simulink model "sampleModel1928_2_sub_sub"  (R2023a)
settings: Solver=VariableStepAuto  StartTime=0.0  StopTime=10.0  RelTol=1e-3
libraries: hdlsllib x7, simulink x2
settings Model: Creator=user1  LastModifiedBy=user1

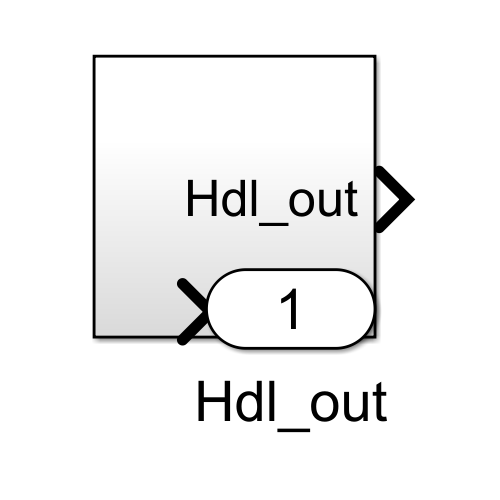
[thumbnail: Simulink's stored preview of the top-level diagram]
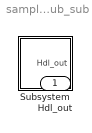
== system sampleModel1928_2_sub_sub ==
  Subsystem : Subsystem
  Hdl_out : Outport  OutDataTypeStr=uint8

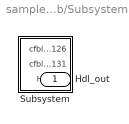
== system sampleModel1928_2_sub_sub/Subsystem ==
  Subsystem : Subsystem
  Hdl_out : Outport  OutDataTypeStr=uint8

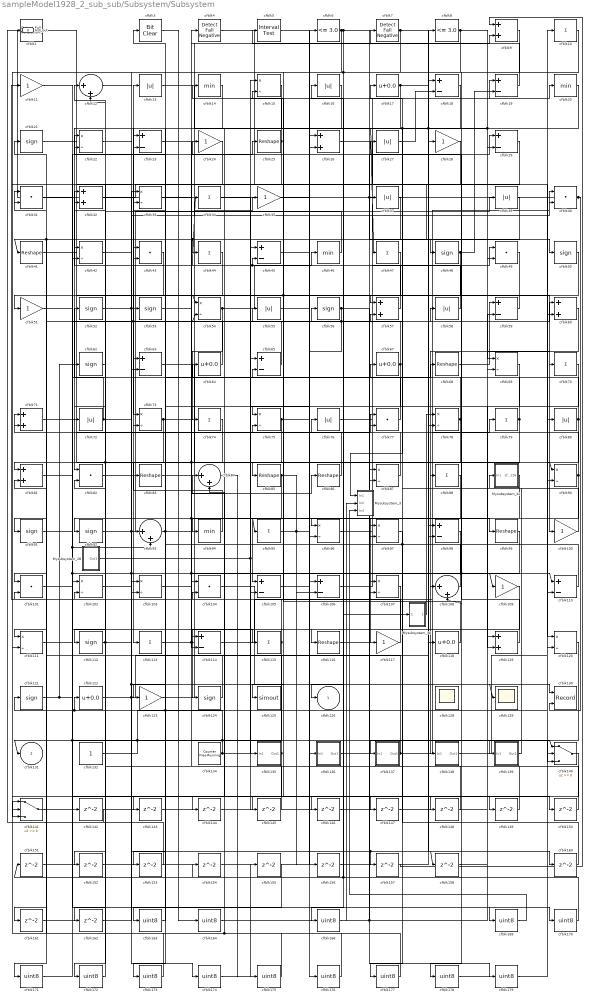
== system sampleModel1928_2_sub_sub/Subsystem/Subsystem ==
  Mysubsystem_28 : Subsystem  TreatAsAtomicUnit=on  RTWFcnName=Mysubsystem_28
      settings: RTWFcnNameOpts=User specified  RTWFileNameOpts=Use function name
  Mysubsystem_3 : Subsystem  TreatAsAtomicUnit=on  RTWFcnName=Mysubsystem_3
      settings: RTWFcnNameOpts=User specified  RTWFileNameOpts=Use function name
  Mysubsystem_38 : Subsystem  TreatAsAtomicUnit=on  RTWFcnName=Mysubsystem_38
      settings: RTWFcnNameOpts=User specified  RTWFileNameOpts=Use function name
  Mysubsystem_42 : Subsystem  TreatAsAtomicUnit=on  RTWFcnName=Mysubsystem_42
      settings: RTWFcnNameOpts=User specified  RTWFileNameOpts=Use function name
  cfblk1 : hdlsllib/Logic and Bit Operations/Detect Fall Nonpositive  vinit=0  OutDataTypeStr=uint8
  cfblk{10,34,44,47,70,74,79,88,95,113,115} (11 alike) : Sum  Inputs=+  OutDataTypeStr=uint8
  cfblk{11,24,28,35,51,100,109,117,123} (9 alike) : Gain  OutDataTypeStr=uint8
  cfblk{31,40,43,49,77,82,101,104} (8 alike) : DotProduct  OutDataTypeStr=uint8
  cfblk{15,22,33,42,54,69,73,75,78,87,90,96..97,102..103,107,111,120} (18 alike) : Product  Inputs=*/  OutDataTypeStr=uint8  RndMeth=Zero  SaturateOnIntegerOverflow=on
  cfblk{18..19,23,29,45,59,63,65,98,105..106,110,114} (13 alike) : Sum  Inputs=+-  OutDataTypeStr=uint8
  cfblk{12,84,93,108} (4 alike) : Sum  Inputs=|++  OutDataTypeStr=uint8
  cfblk{21,48,50,52..53,56,62,91..92,112,121,124} (12 alike) : Signum
  cfblk{25,41,68,83,85..86,99,116} (8 alike) : Reshape
  cfblk{17,64,67,118,122} (5 alike) : Bias  Bias=0.0  SaturateOnIntegerOverflow=off
  cfblk{9,26,32,57,60,71,81,119} (8 alike) : Sum  OutDataTypeStr=uint8
  cfblk125 : ToWorkspace  VariableName=simout  SaveFormat=Timeseries  SampleTime=-1
  cfblk128 : Scope
      settings: Floating=on
  cfblk129 : Scope
  cfblk{13,16,27,37,39,55,58,72,76,80} (10 alike) : Abs  OutDataTypeStr=uint8  SaturateOnIntegerOverflow=off
  cfblk130 : Record  FileSettingsInternal="{\"entries\":[{\"content\":{\"excelSettings\":{\"content\":{},\"type\":\"Streamout.ExcelSettings\"}},\"type\":\"Streamout.FileSettingStorage\",\"uuid\":\"\"}],\"packageUris\":[\"http:\\/\\/schema.mathworks.com\\/mf0\\/streamout_blocks\\/R2020a\"],\"version\":\"1.0\"}"  Layout=[1 1]  SignalsInternal="{\"entries\":[{\"content\":{\"signals\":[{\"content\":{\"blockPath\":[],\"dimensions\":[1],\"domain\":\"\",\"lineColor\":\"#a2142f\",\"plots\":[1],\"port\":1,\"signalID\":52207,\"signalName\":\"cfblk34\"},\"type\":\"RecordBlkView.Signal\",\"uuid\":\"\"},{\"content\":{\"blockPath\":[],\"dimensions\":[1],\"domain\":\"\",\"lineColor\":\"#139fff\",\"plots\":[1],\"port\":2,\"signalID\":52210,\"signalName\":\"cfblk40\"},\"type\":\"RecordBlkView.Signal\",\"uuid\":\"\"}]},\"type\":\"RecordBlkView.InputSignals\",\"uuid\":\"\"}],\"packageUris\":[\"http:\\/\\/schema.mathworks.com\\/mf0\\/streamout_blocks\\/R2020a\"],\"version\":\"1.0\"}"  VisualizationBindings="{\"xyplotplugin\":{\"info\":[{\"series\":[{\"bindingParametersList\":[{\"parameter\":\"X-Axis\",\"signalID\":52207,\"signalName\":\"cfblk34\"},{\"parameter\":\"Y-Axis\",\"signalID\":52210,\"signalName\":\"cfblk40\"}],\"seriesID\":26218}],\"subplotID\":1}]}}"  CompatibilityTag=XY  st=-1
  cfblk132 : Constant  OutDataTypeStr=uint8  SampleTime=-1
  cfblk134 : hdlsllib/Sources/Counter Free-Running  NumBits=16  tsamp=-1
  cfblk135 : Subsystem
      settings: LibrarySourceBlock=|
      | hdlsllib/Ports &
      | Subsystems/Subsystem
  cfblk136 : Subsystem
      settings: LibrarySourceBlock=|
      | hdlsllib/Ports &
      | Subsystems/Subsystem
  cfblk137 : Subsystem
      settings: LibrarySourceBlock=|
      | hdlsllib/Ports &
      | Subsystems/Subsystem
  cfblk138 : Subsystem
      settings: LibrarySourceBlock=|
      | hdlsllib/Ports &
      | Subsystems/Subsystem
  cfblk139 : Subsystem
      settings: LibrarySourceBlock=|
      | hdlsllib/Ports &
      | Subsystems/Subsystem
  cfblk{14,20,46,94} (4 alike) : MinMax  OutDataTypeStr=uint8
  cfblk140 : Switch  OutDataTypeStr=uint8  SaturateOnIntegerOverflow=off  InputSameDT=off
  cfblk141 : Switch  OutDataTypeStr=uint8  SaturateOnIntegerOverflow=off  InputSameDT=off
  cfblk{142..158,160..162} (20 alike) : Delay  SampleTime=1
  cfblk{163..164,166,169..179} (14 alike) : DataTypeConversion  OutDataTypeStr=uint8  SaturateOnIntegerOverflow=off  RndMeth=Floor
  cfblk3 : simulink/Logic and Bit Operations/Bit Clear  iBit=0
      settings: LibrarySourceBlock=|
      | hdlsllib/Logic and Bit
      | Operations/Bit Clear
  cfblk4 : hdlsllib/Logic and Bit Operations/Detect Fall Negative  vinit=0  OutDataTypeStr=uint8
  cfblk5 : hdlsllib/Logic and Bit Operations/Interval Test  IntervalClosedRight=on  uplimit=0.5  IntervalClosedLeft=on  lowlimit=-0.5  OutDataTypeStr=uint8
  cfblk6 : hdlsllib/Logic and Bit Operations/Compare To Constant  relop=<=  const=3.0  OutDataTypeStr=uint8
  cfblk7 : hdlsllib/Logic and Bit Operations/Detect Fall Negative  vinit=0  OutDataTypeStr=uint8
  cfblk8 : hdlsllib/Logic and Bit Operations/Compare To Constant  relop=<=  const=3.0  OutDataTypeStr=uint8
  cfblk126 : Outport  OutDataTypeStr=uint8  VectorParamsAs1DForOutWhenUnconnected=off
  cfblk131 : Outport  Port=2  OutDataTypeStr=uint8  VectorParamsAs1DForOutWhenUnconnected=off
  Hdl_out : Outport  Port=3  OutDataTypeStr=uint8
  wires:
  Mysubsystem_42/1(cfblk126) -> cfblk126/1
  cfblk139/1(Out1) -> Mysubsystem_42/1(In1)
  Mysubsystem_38/1(Out1) -> cfblk78/1
  Mysubsystem_28/1(Out1) -> cfblk106/1, cfblk135/1(In1)
  cfblk169/1 -> Mysubsystem_3/3(In3)
  cfblk166/1 -> Mysubsystem_3/2(In2)
  cfblk179/1 -> cfblk10/1
  cfblk178/1 -> cfblk120/2
  cfblk10/1 -> cfblk178/1
  cfblk177/1 -> cfblk84/2
  cfblk120/1 -> cfblk177/1
  cfblk176/1 -> cfblk84/1
  cfblk5/1 -> cfblk176/1
  cfblk175/1 -> cfblk154/1, cfblk121/1
  cfblk174/1 -> cfblk155/1
  cfblk42/1 -> cfblk174/1
  cfblk173/1 -> cfblk141/1
  cfblk155/1 -> cfblk173/1
  cfblk172/1 -> cfblk102/2
  cfblk62/1 -> cfblk172/1
  cfblk171/1 -> cfblk102/1
  cfblk170/1 -> cfblk151/1, cfblk76/1
  cfblk164/1 -> cfblk69/2, cfblk87/2
  cfblk163/1 -> cfblk3/1
  cfblk140/1 -> cfblk163/1
  cfblk162/1 -> cfblk33/1
  cfblk161/1 -> cfblk103/2
  cfblk160/1 -> cfblk57/2
  cfblk158/1 -> cfblk59/2
  cfblk157/1 -> cfblk9/1
  cfblk156/1 -> cfblk97/2
  cfblk154/1 -> cfblk98/2
  cfblk153/1 -> cfblk31/2
  cfblk152/1 -> cfblk26/2
  cfblk151/1 -> cfblk93/1
  cfblk150/1 -> cfblk87/1
  cfblk105/1 -> cfblk150/1
  cfblk149/1 -> cfblk104/1
  cfblk148/1 -> cfblk82/2
  cfblk147/1 -> cfblk18/1
  cfblk11/1 -> cfblk147/1
  cfblk146/1 -> cfblk119/1
  cfblk145/1 -> cfblk65/1
  cfblk107/1 -> cfblk145/1
  cfblk144/1 -> cfblk45/1
  cfblk143/1 -> cfblk15/1
  cfblk142/1 -> cfblk1/1
  cfblk111/1 -> cfblk142/1
  cfblk45/1 -> cfblk97/1
  cfblk54/1 -> cfblk46/1, cfblk74/1
  cfblk20/1 -> cfblk83/1, cfblk29/2
  cfblk35/1 -> cfblk99/1
  cfblk115/1 -> cfblk101/2, cfblk161/1
  cfblk116/1 -> cfblk68/1
  cfblk104/1 -> cfblk136/1(In1)
  cfblk88/1 -> cfblk107/1
  cfblk82/1 -> cfblk26/1
  cfblk46/1 -> cfblk22/1
  cfblk110/1 -> cfblk27/1, cfblk22/2
  cfblk124/1 -> cfblk71/2
  cfblk33/1 -> cfblk96/1, cfblk90/1
  cfblk53/1 -> cfblk114/1
  cfblk77/1 -> cfblk16/1
  cfblk22/1 -> cfblk107/2, cfblk148/1
  cfblk25/1 -> cfblk111/2, cfblk14/1
  cfblk99/1 -> cfblk108/2, cfblk114/2
  cfblk55/1 -> cfblk108/1
  cfblk59/1 -> cfblk57/1
  cfblk73/1 -> cfblk118/1, cfblk91/1
  cfblk109/1 -> cfblk124/1
  cfblk95/1 -> cfblk6/1, cfblk156/1
  cfblk49/1 -> cfblk54/1, cfblk85/1
  cfblk135/1(Out1) -> cfblk141/2, cfblk12/2
  cfblk3/1 -> cfblk164/1
  cfblk121/1 -> cfblk67/1, cfblk62/1
  cfblk67/1 -> cfblk43/2, cfblk153/1
  cfblk138/1(Out1) -> cfblk110/2
  cfblk84/1 -> cfblk175/1
  cfblk13/1 -> cfblk49/2
  cfblk63/1 -> cfblk98/1
  cfblk26/1 -> cfblk69/1
  cfblk24/1 -> cfblk123/1
  cfblk39/1 -> cfblk42/2, cfblk44/1
  cfblk80/1 -> cfblk23/2, cfblk90/2
  cfblk37/1 -> cfblk41/1, cfblk81/1
  cfblk44/1 -> cfblk72/1
  cfblk117/1 -> cfblk104/2
  cfblk112/1 -> cfblk53/1, cfblk12/1
  cfblk23/1 -> cfblk95/1, cfblk105/2
  cfblk50/1 -> cfblk101/1
  cfblk60/1 -> cfblk88/1
  cfblk132/1 -> cfblk140/1, cfblk80/1
  cfblk70/1 -> cfblk94/1
  cfblk118/1 -> cfblk65/2
  cfblk8/1 -> cfblk63/2, cfblk70/1
  cfblk1/1 -> cfblk103/1
  cfblk90/1 -> cfblk56/1, cfblk162/1
  cfblk103/1 -> cfblk9/2, cfblk109/1
  cfblk68/1 -> cfblk59/1
  cfblk100/1 -> cfblk17/1
  cfblk19/1 -> cfblk5/1
  cfblk136/1(Out1) -> cfblk37/1, cfblk29/1
  cfblk9/1 -> cfblk116/1
  cfblk18/1 -> Mysubsystem_3/1(In1), cfblk47/1, cfblk78/2
  cfblk28/1 -> cfblk42/1
  cfblk76/1 -> cfblk49/1
  cfblk64/1 -> cfblk32/2
  cfblk69/1 -> cfblk119/2
  cfblk47/1 -> cfblk63/1
  cfblk43/1 -> cfblk111/1
  cfblk101/1 -> cfblk60/1
  cfblk65/1 -> cfblk43/1, cfblk31/1
  cfblk91/1 -> cfblk110/1, cfblk115/1
  cfblk106/1 -> cfblk58/1
  cfblk51/1 -> cfblk93/2, cfblk169/1
  cfblk96/1 -> cfblk20/1
  cfblk12/1 -> cfblk129/1, cfblk149/1
  cfblk56/1 -> cfblk96/2, cfblk54/2, cfblk179/1
  cfblk29/1 -> cfblk92/1
  cfblk87/1 -> cfblk21/1
  cfblk31/1 -> cfblk140/2, cfblk143/1
  cfblk58/1 -> cfblk32/1
  cfblk108/1 -> cfblk23/1
  cfblk98/1 -> cfblk117/1
  cfblk114/1 -> cfblk40/1
  cfblk83/1 -> cfblk4/1
  cfblk41/1 -> cfblk100/1
  cfblk81/1 -> cfblk25/1
  cfblk7/1 -> Mysubsystem_38/1(In1), cfblk125/1, cfblk160/1
  cfblk15/1 -> cfblk73/1
  cfblk74/1 -> cfblk112/1
  cfblk40/1 -> cfblk130/2, Hdl_out/1
  cfblk94/1 -> cfblk13/1
  cfblk97/1 -> cfblk137/1(In1)
  cfblk34/1 -> cfblk130/1
  cfblk17/1 -> cfblk60/2, cfblk144/1
  cfblk141/1 -> cfblk28/1
  cfblk72/1 -> cfblk52/1, cfblk64/1
  cfblk71/1 -> cfblk75/2
  cfblk85/1 -> cfblk105/1, cfblk106/2
  cfblk79/1 -> cfblk15/2, cfblk166/1
  cfblk75/1 -> cfblk152/1, cfblk171/1, cfblk139/1(In1)
  cfblk4/1 -> cfblk120/1
  cfblk57/1 -> cfblk34/1, cfblk45/2
  cfblk86/1 -> cfblk71/1
  cfblk92/1 -> cfblk39/1, cfblk77/2
  cfblk122/1 -> cfblk8/1, cfblk140/3
  cfblk21/1 -> cfblk138/1(In1)
  cfblk78/1 -> cfblk113/1, cfblk55/1
  cfblk16/1 -> cfblk75/1
  cfblk6/1 -> cfblk48/1, cfblk146/1, cfblk141/3
  cfblk14/1 -> cfblk82/1
  cfblk93/1 -> cfblk11/1, cfblk86/1
  cfblk119/1 -> cfblk24/1
  cfblk48/1 -> cfblk51/1, cfblk19/2
  cfblk52/1 -> cfblk157/1, cfblk158/1, cfblk40/2
  cfblk102/1 -> cfblk170/1
  cfblk113/1 -> cfblk7/1, cfblk77/1
  cfblk27/1 -> cfblk18/2
  cfblk32/1 -> cfblk50/1
  cfblk123/1 -> cfblk35/1
  cfblk137/1(Out1) -> cfblk79/1, cfblk33/2
  cfblk134/1 -> cfblk122/1, cfblk81/2, cfblk73/2, cfblk131/1, cfblk19/1

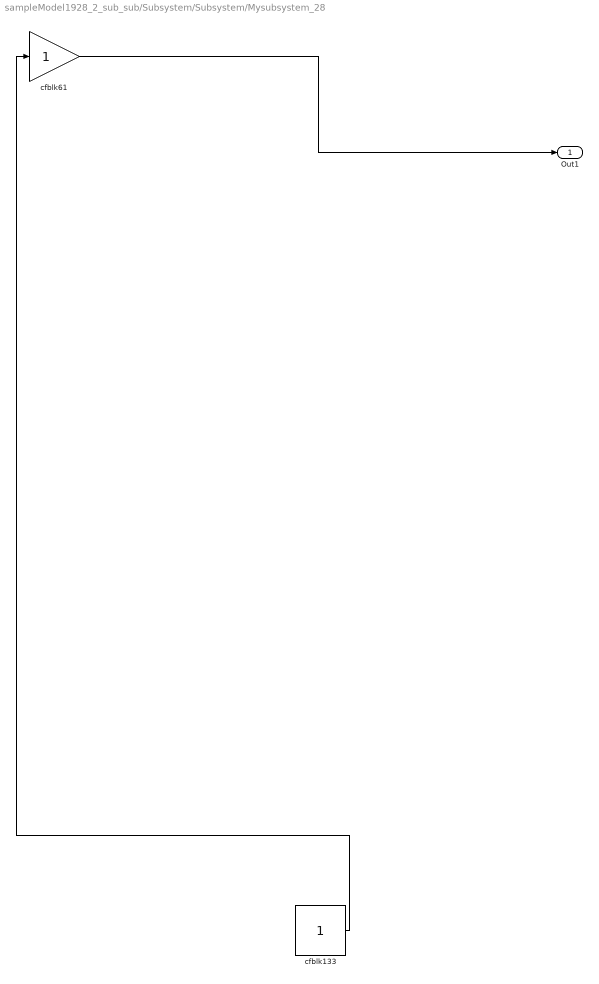
== system sampleModel1928_2_sub_sub/Subsystem/Subsystem/Mysubsystem_28 ==
  cfblk133 : Constant  SampleTime=-1
  cfblk61 : Gain
  Out1 : Outport
  wires:
  cfblk133/1 -> cfblk61/1
  cfblk61/1 -> Out1/1

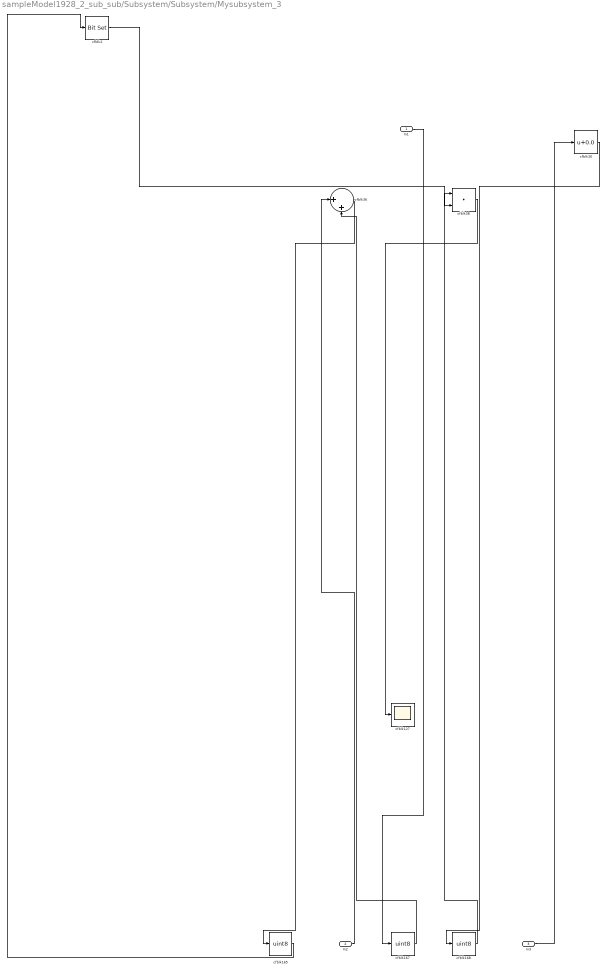
== system sampleModel1928_2_sub_sub/Subsystem/Subsystem/Mysubsystem_3 ==
  In1 : Inport
  In2 : Inport  Port=2
  In3 : Inport  Port=3
  cfblk127 : Scope
  cfblk165 : DataTypeConversion  OutDataTypeStr=uint8  SaturateOnIntegerOverflow=off  RndMeth=Floor
  cfblk167 : DataTypeConversion  OutDataTypeStr=uint8  SaturateOnIntegerOverflow=off  RndMeth=Floor
  cfblk168 : DataTypeConversion  OutDataTypeStr=uint8  SaturateOnIntegerOverflow=off  RndMeth=Floor
  cfblk2 : simulink/Logic and Bit Operations/Bit Set  iBit=0
      settings: LibrarySourceBlock=|
      | hdlsllib/Logic and Bit
      | Operations/Bit Set
  cfblk30 : Bias  Bias=0.0  SaturateOnIntegerOverflow=off
  cfblk36 : Sum  Inputs=|++
  cfblk38 : DotProduct  OutDataTypeStr=Inherit: Inherit via internal rule
  wires:
  cfblk167/1 -> cfblk36/2
  cfblk2/1 -> cfblk38/2
  In2/1 -> cfblk36/1
  cfblk168/1 -> cfblk38/1
  cfblk30/1 -> cfblk168/1
  cfblk36/1 -> cfblk165/1
  cfblk38/1 -> cfblk127/1
  cfblk165/1 -> cfblk2/1
  In3/1 -> cfblk30/1
  In1/1 -> cfblk167/1

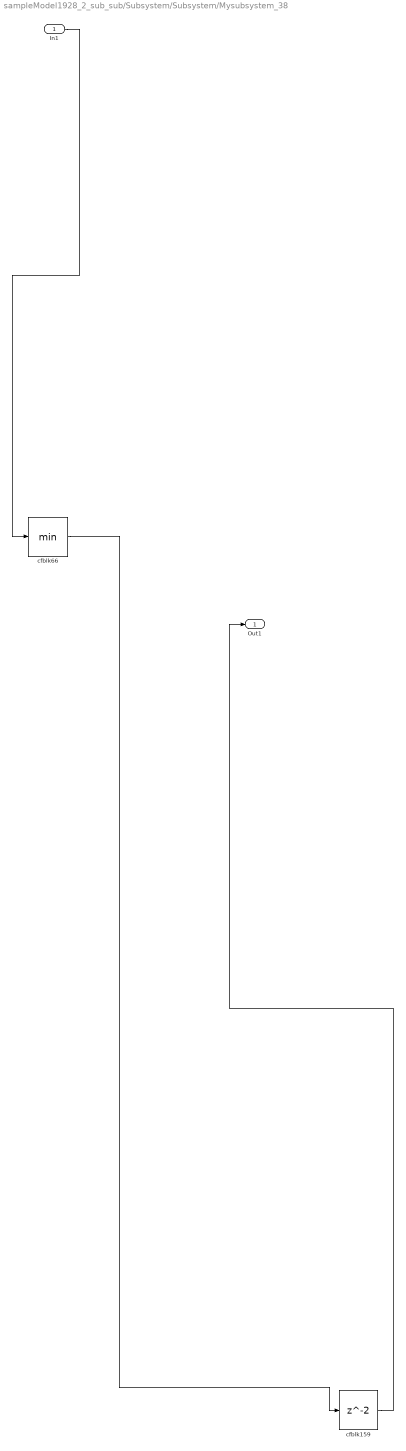
== system sampleModel1928_2_sub_sub/Subsystem/Subsystem/Mysubsystem_38 ==
  In1 : Inport
  cfblk159 : Delay  SampleTime=1
  cfblk66 : MinMax
  Out1 : Outport
  wires:
  cfblk66/1 -> cfblk159/1
  In1/1 -> cfblk66/1
  cfblk159/1 -> Out1/1

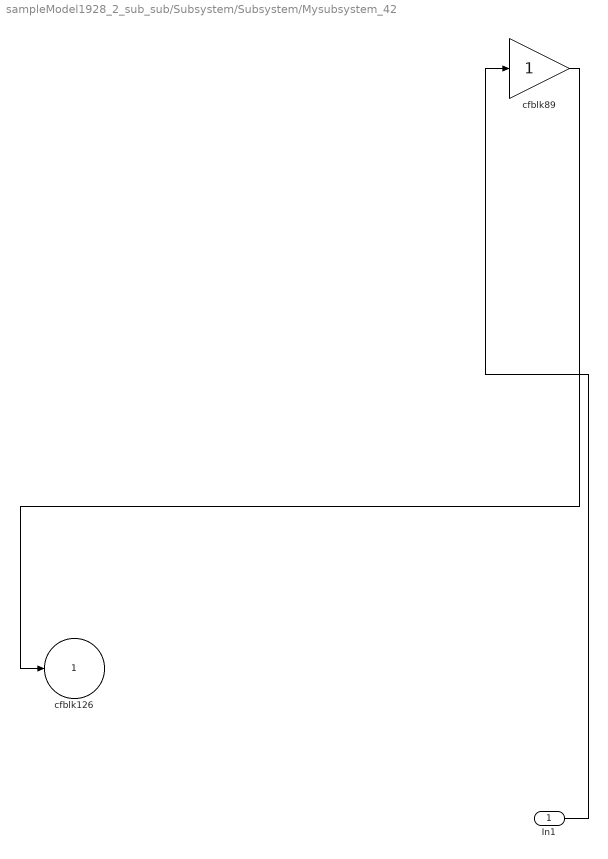
== system sampleModel1928_2_sub_sub/Subsystem/Subsystem/Mysubsystem_42 ==
  In1 : Inport
  cfblk89 : Gain
  cfblk126 : Outport  VectorParamsAs1DForOutWhenUnconnected=off
  wires:
  cfblk89/1 -> cfblk126/1
  In1/1 -> cfblk89/1

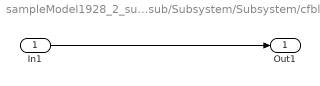
== system sampleModel1928_2_sub_sub/Subsystem/Subsystem/cfblk135 ==
  In1 : Inport
  Out1 : Outport
  wires:
  In1/1 -> Out1/1

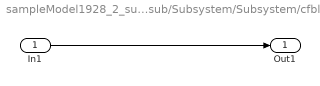
== system sampleModel1928_2_sub_sub/Subsystem/Subsystem/cfblk136 ==
  In1 : Inport
  Out1 : Outport
  wires:
  In1/1 -> Out1/1

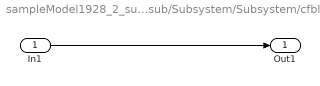
== system sampleModel1928_2_sub_sub/Subsystem/Subsystem/cfblk137 ==
  In1 : Inport
  Out1 : Outport
  wires:
  In1/1 -> Out1/1

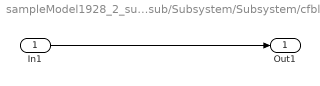
== system sampleModel1928_2_sub_sub/Subsystem/Subsystem/cfblk138 ==
  In1 : Inport
  Out1 : Outport
  wires:
  In1/1 -> Out1/1

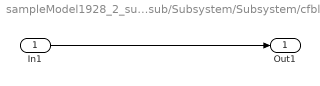
== system sampleModel1928_2_sub_sub/Subsystem/Subsystem/cfblk139 ==
  In1 : Inport
  Out1 : Outport
  wires:
  In1/1 -> Out1/1
